simulink model "SimplePlungerMdl"  (R2022b)
settings: Solver=VariableStepAuto  StartTime=0.0  StopTime=10  MaxStep=.001  RelTol=1e-4
values from neighbouring files (symbols this model uses):
  x_init = x0 + 1e-3    (= 0.006)    [SimpleSolenoid.m]
undefined symbols (not defined in the file or in its folder): sigbuilder_block
libraries: fl_lib x5, nesl_utility x4, ee_lib x1
settings Model: PacingRate=0.630000  Creator=Sajjad  LastModifiedBy=Sajjad

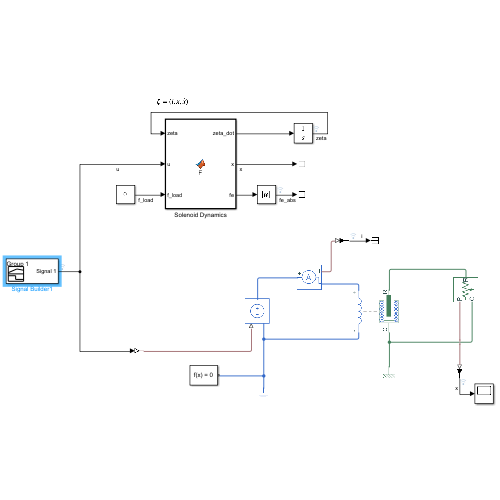
[thumbnail: Simulink's stored preview of the top-level diagram]
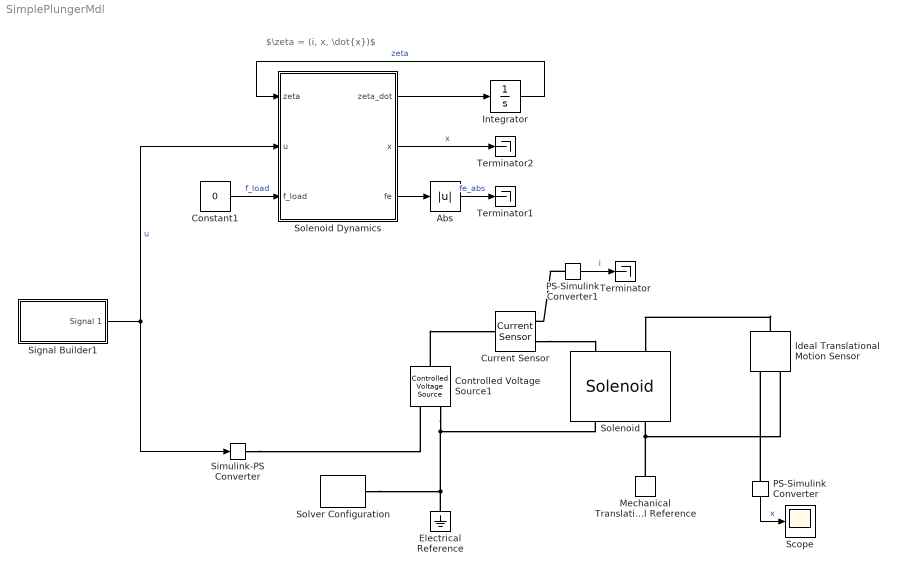
== system SimplePlungerMdl ==
  note: $\zeta = (i, x, \dot{x})$
  Abs : Abs  SaturateOnIntegerOverflow=off
  Constant1 : Constant  Value=0
  Controlled Voltage Source1 : fl_lib/Electrical/Electrical Sources/Controlled Voltage Source
  Current Sensor : fl_lib/Electrical/Electrical Sensors/Current Sensor
  Electrical Reference : fl_lib/Electrical/Electrical Elements/Electrical Reference
  Ideal Translational Motion Sensor : fl_lib/Mechanical/Mechanical Sensors/Ideal Translational Motion Sensor  reference=foundation.enum.MeasurementReference.difference  acceleration_port=false  velocity_port=false  position_port=true  offset=x_init m
      settings: InternalSimscapePortConfiguration="{\"Bottom\":[],\"Left\":[{\"id\":\"R\",\"label\":\"R\",\"type\":\"foundation.mechanical.translational.translational\"}],\"Right\":[{\"id\":\"C\",\"label\":\"C\",\"type\":\"foundation.mechanical.translational.translational\"},{\"id\":\"P\",\"label\":\"P\",\"type\":\"output\"}],\"Top\":[]}"
  Integrator : Integrator  InitialCondition=[0, x_init, 0]
  Mechanical Translational Reference : fl_lib/Mechanical/Translational Elements/Mechanical Translational Reference
  PS-Simulink Converter : nesl_utility/PS-Simulink Converter  PhysicalDomain=network_engine_domain  SubClassName=ps_output  LeftPortType=input  RightPortType=output  PseudoPeriodic=off  Frequencies=[]  VectorFormat=inherit  Unit=inherit  AffineConversion=off
  PS-Simulink Converter1 : nesl_utility/PS-Simulink Converter  PhysicalDomain=network_engine_domain  SubClassName=ps_output  LeftPortType=input  RightPortType=output  PseudoPeriodic=off  Frequencies=[]  VectorFormat=inherit  Unit=inherit  AffineConversion=off
  Scope : Scope
  Signal Builder1 : Subsystem  Tag=STV Subsys  LoadFcn=sigbuilder_block('load',[157.2 146.4 550.8 400.2 ]);  StartFcn=sigbuilder_block('start');  StopFcn=sigbuilder_block('stop');  ClipboardFcn=sigbuilder_block('clipboard');  mask(Sigbuilder block){tuvar=[0:10]}
      mask help: Simulink:masks:SigbuilderBlock_MD
      mask init:
      | if ~strcmp(get_param(bdroot(gcbh),'SimulationStatus'),'stopped') tuvar = sigbuilder_block('maskInit'); end
      settings: CopyFcn=sigbuilder_block('copy');  DeleteFcn=sigbuilder_block('delete');  ModelCloseFcn=sigbuilder_block('modelClose');  PreSaveFcn=sigbuilder_block('preSave');  PauseFcn=sigbuilder_block('pause');  ContinueFcn=sigbuilder_block('continue');  NameChangeFcn=sigbuilder_block('namechange');  OpenFcn=sigbuilder_block('open',[256.8 151.8 550.8 400.2 ]);  CloseFcn=sigbuilder_block('close');
      mask Display: plot(0, 0, 100, 100,[2, 2, 32, 32, 2], [68, 8, 8, 68, 68],[32, 2], [38, 38], [32, 19, 2],[53, 60, 44], [32, 17, 17, 2],[16, 16, 31, 31]);txt = getActiveGroup(gcbh);text(2, 100, txt,'verticalAlignment', 'top');
  Simulink-PS Converter : nesl_utility/Simulink-PS Converter  PhysicalDomain=network_engine_domain  SubClassName=ps_input  LeftPortType=input  RightPortType=output  PseudoPeriodic=off  Frequencies=[]  NoiseDistribution=none  NoiseParameters=[]  Unit=1  AffineConversion=off  FilteringAndDerivatives=provide  SimscapeFilterOrder=1  InputFilterTimeConstant=0.001  UdotUserProvided=0
  Solenoid : ee_lib/Electromechanical/Mechatronic Actuators/Solenoid  motionDirection=ee.enum.actuators.solenoidDirection.towards  F12=[7.5, .75] N  X12=[1, 5] mm  Vdc=50 V  Imax=0.05 A  K=200 N/m  Xzero=5 mm  lam=1 N*s/m  Mass=0.05 kg  Xmax=Inf mm  K_endstop=1e6 N/m  D_endstop=500 N*s/m  i_specify=off  i_priority=High  i=0 A  i_nominal_specify=off  i_nominal_unit=A  i_nominal_value=1  x_specify=on  x_priority=High  x=x_init m  x_nominal_specify=off  x_nominal_unit=mm  x_nominal_value=1  vel_specify=off  vel_priority=None  vel=0 mm/s  vel_nominal_specify=off  vel_nominal_unit=mm/s  vel_nominal_value=1  F_specify=off  F_priority=None  F=0 N  F_nominal_specify=off  F_nominal_unit=N  F_nominal_value=1  v_L_specify=off  v_L_priority=None  v_L=0 V  v_L_nominal_specify=off  v_L_nominal_unit=V  v_L_nominal_value=1  magnetic_force_specify=off  magnetic_force_priority=None  magnetic_force=0 N  magnetic_force_nominal_specify=off  magnetic_force_nominal_unit=N  magnetic_force_nominal_value=1  alpha=3.93e-3 1/K  Tmeas=25 degC  thermal_mass=100 J/K  temperature_specify=off  temperature_priority=High  temperature=25 degC  temperature_nominal_specify=off  temperature_nominal_unit=degC  temperature_nominal_value=1  Q_specify=off  Q_priority=None  Q=0 W  Q_nominal_specify=off  Q_nominal_unit=W  Q_nominal_value=1
      settings: InternalSimscapePortConfiguration="{\"Bottom\":[],\"Left\":[{\"id\":\"p\",\"label\":\"+\",\"type\":\"foundation.electrical.electrical\"},{\"id\":\"R\",\"label\":\"R\",\"type\":\"foundation.mechanical.translational.translational\"}],\"Right\":[{\"id\":\"n\",\"label\":\"-\",\"type\":\"foundation.electrical.electrical\"},{\"id\":\"C\",\"label\":\"C\",\"type\":\"foundation.mechanical.translational.translational\"}],\"Top\":[]}"
  Solenoid Dynamics : MATLAB Function  TreatAsAtomicUnit=on
  Solver Configuration : nesl_utility/Solver Configuration  PhysicalDomain=network_engine_domain  SubClassName=solver  LeftPortType=input  RightPortType=generic  Tones=[]  Harmonics=[]  SimulateNoise=off  Profile=off  UseLocalSampling=off  EnableSwitchedLinearOptims=on  FrequencyDomain=off  UseCCode=off  RelTol=0.001  AbsTol=0.001  MinStep=1e-09  ToWorkspace=off  RevertToSquareIcSolve=off  NumHomotopyIterations=100  PhasorMode=off  PhasorModeNumHarmonics=1  ConsistencySolver=NEWTON_XTOL_AFTER_FTOL  IndexReductionMethod=DerivativeReplacement  DoDC=off  ResidualTolerance=1e-09  ConsistencyTolSource=GLOBAL  ConsistencyAbsTol=0.001  ConsistencyRelTol=0.001  ConsistencyTolFactor=0.001  UseLocalSolver=off  LocalSolverChoice=NE_BACKWARD_EULER_ADVANCER  ResolveIndetEquations=on  FunctionEvalNumThread=1  LocalSolverSampleTime=0.001  DoFixedCost=off  MaxNonlinIter=3  MaxModeIter=2  ComputeImpulses=off  ImpulseIterations=2  LinearAlgebra=auto  LinearAlgebraNumThread=0  EquationFormulation=NE_TIME_EF  DelaysMemoryBudget=1024  AutomaticFiltering=on  FilteringTimeConstant=0.001  PartitionStorageMethod=AS_NEEDED  PartitionMemoryBudget=1024  PartitionMethod=ROBUST
  Terminator : Terminator
  Terminator1 : Terminator
  Terminator2 : Terminator
  wires:
  Signal Builder1/1(Signal 1) -> Solenoid Dynamics/2(u), Simulink-PS Converter/1  "u"
  Solenoid Dynamics/1(zeta_dot) -> Integrator/1
  Integrator/1 -> Solenoid Dynamics/1(zeta)  "zeta"
  PS-Simulink Converter/1 -> Scope/1  "x"
  PS-Simulink Converter1/1 -> Terminator/1  "i"
  Solenoid Dynamics/3(fe) -> Abs/1
  Abs/1 -> Terminator1/1  "fe_abs"
  Solenoid Dynamics/2(x) -> Terminator2/1  "x"
  Constant1/1 -> Solenoid Dynamics/3(f_load)  "f_load"
  connections:
  Controlled Voltage Source1/LConn1 -- Current Sensor/LConn1
  Solver Configuration/RConn1 -- Controlled Voltage Source1/RConn2 -- Solenoid/RConn1 -- Electrical Reference/LConn1
  Mechanical Translational Reference/LConn1 -- Ideal Translational Motion Sensor/RConn1 -- Solenoid/RConn2
  Ideal Translational Motion Sensor/LConn1 -- Solenoid/LConn2
  PS-Simulink Converter/LConn1 -- Ideal Translational Motion Sensor/RConn2
  Current Sensor/RConn2 -- Solenoid/LConn1
  PS-Simulink Converter1/LConn1 -- Current Sensor/RConn1
  Simulink-PS Converter/RConn1 -- Controlled Voltage Source1/RConn1

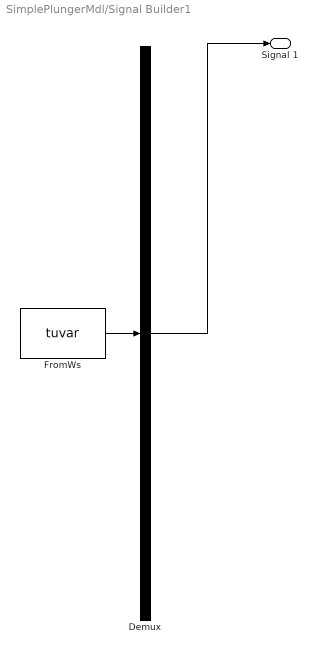
== system SimplePlungerMdl/Signal Builder1 ==
  Demux : Demux  Tag=STV Demux  Outputs=1
      settings: DisplayOption=none
  FromWs : FromWorkspace  Tag=STV FromWs  VariableName=tuvar
      SigBuilderData=|
      | common.afterFinalStr = 'Extrapolate'
      | common.sampleTime = 0
      | dataSet.timeRange = [0 10]
      | dataSet.name = 'Group 1'
      | sbobj.Groups.Name = 'Group 1'
      | sbobj.Groups.Signals.Name = 'Signal 1'
      | sbobj.Groups.Signals.XData = [0 2 2 4 4 10]
      | sbobj.Groups.Signals.YData = [0 0 15 15 0 0]
  Signal 1 : Outport  Tag=STV Outport
  wires:
  Demux/1 -> Signal 1/1
  FromWs/1 -> Demux/1

== matlab function SimplePlungerMdl/Solenoid Dynamics ==
  data: zeta input; u input; f_load input; zeta_dot output; x output; params parameter; fe output
function [zeta_dot, x, fe] = F(zeta, u, f_load, params)
% zeta: state variables
% zeta_dot: state derivatives
% u: input signal: applied voltage on the electrical circuit
% x0: resting position of the plunger with the spring at relaxed state

% zeta = [i, x, x_dot]
% i: current
% x: air-gap length = plunger position
% x_dot: plunger velocity

zeta_dot = zeros(1,3);

i = zeta(1);
x = zeta(2);
x_dot = zeta(3);

alpha0 = params.alpha0;
beta0 = params.beta0;

L = 1 ./ (alpha0 + beta0 .* x);
Lp = -beta0 ./ ((alpha0 + beta0 .* x).^2);
fe = 1/2 * i^2 * Lp;

zeta_dot(1) = 1/(params.l + L) * (u - params.r*i - Lp*x_dot*i);
zeta_dot(2) = x_dot;
zeta_dot(3) = 1/params.m * (f_load + fe - params.k * (x-params.x0) - params.c * x_dot);

end
